simulink model "Exercise11"  (Simulink 7.2)
settings: Solver=ode45  StartTime=0.0  StopTime=2000.0  RelTol=1e-3
undefined symbols (not defined in the file): des_figposition
libraries: simeventssink1 x2, simeventsgenerators1 x2, simeventstiming1 x2, simeventsqueue1 x1, simeventsserver1 x1
settings Model: Creator=inderjot  LastModifiedBy=inderjot
settings SimEventsCC: propLogEventsScheduled=0  propLogEventsExecuted=0  propLogDepartureEvents=0  propDisplayEventCalendar=0  propDiagAttribOutput=1  propDiagFcnCallOutput=1  propDiagStatOutput=0

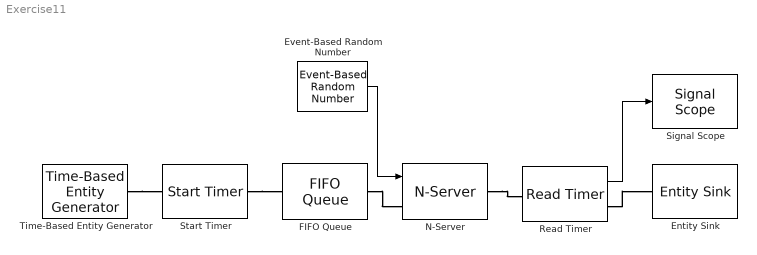
== system Exercise11 ==
  Entity Sink : simeventssink1/Entity Sink  Priority=1  SystemSampleTime=-1  AvailableForArrivals=on  StatNumberArrived=Off
  Event-Based Random Number : simeventsgenerators1/Signal Generators/Event-Based Random Number  SystemSampleTime=-1  distribution=Exponential  meanExp=5  minUnif=1  maxUnif=1  pOneBern=0.25  pSuccessBino=0.5  numTrialBino=1  meanNorm=0  stdNorm=1  minTri=1  maxTri=3  modeTri=2  thresholdLogn=0  scaleLogn=1  shapeLogn=1  pSuccessGeo=0.5  meanPoiss=1  thresholdLogl=0  scaleLogl=1  thresholdGam=0  scaleGam=1  shapeGam=1  minBeta=0  maxBeta=1  shape1Beta=1  shape2Beta=1  minUnid=0  maxUnid=1  numValueUnid=2  thresholdWbl=0  scaleWbl=1  shapeWbl=1  valueVecCont=[0 1]  cdfVecCont=[0 1]  valueVecDisc=[0 1]  probVecDisc=[0.5 0.5]  seed=9991125  IsProcessed=on  isConnected=1
  FIFO Queue : simeventsqueue1/FIFO Queue  Priority=1  SystemSampleTime=-1  Capacity=25  EnableTOPort=off  StatNumberDeparted=Off  StatNumberInBlock=Off  StatPendingEntity=Off  StatAverageWait=Off  StatAverageQueueLength=Off  StatNumberTimedout=Off
  N-Server : simeventsserver1/N-Server  Priority=1  SystemSampleTime=-1  NumberOfServers=5  ServiceTimeFrom=Signal port t  ServiceTime=1  AttributeName=ServiceTime  PriorityServiceCompletion=500  EnableTOPort=off  StatNumberDeparted=Off  StatNumberInBlock=Off  StatPendingEntity=Off  StatNumberPending=Off  StatAverageWait=Off  StatUtilization=Off  StatNumberTimedout=Off
  Read Timer : simeventstiming1/Read Timer  Priority=0  SystemSampleTime=-1  TimerTag=T1  TimerModeOption=Error  TimerStop=off  StatNumberDeparted=Off  StatTimerNumberDeparted=Off  StatTimeElapsed=Off  StatAverageTimeElapsed=On
  Signal Scope : simeventssink1/Signal Scope  Priority=1  SystemSampleTime=-1  PlotType=Continuous  InputType=Signal  NumInputs=1  AttributeNameY=Count  XInputOptionSignal=Event time  XInputOptionEntity=Event time  AttributeNameX=Count  EnableEntityOutport=on  XMin=0  XMax=2000  XLimitExceededOption=Keep axis limits unchanged  YLimitExceededOption=Stretch axis limits  AxisGrid=on  AxisLegend=off  LineDisables=""  LineColors=b  LineStyles=-  LineMarkers=.  OpenScopeAtSimStart=on  Title=Average Waiting Time in Queuing System  YLabel=Average Waiting Time  XLabel=Simulation Time  FigurePosition=des_figposition([5 60 25 25])  AxisZoom=off  DataStoreOption=Limited  DataPointsLimit=10000  StatNumberArrived=Off  ShowCountPlotted=off  ShowToolbar=on
      settings: YMin=0  YMax=6
  Start Timer : simeventstiming1/Start Timer  Priority=0  SystemSampleTime=-1  TimerTag=T1  TimerStartedOption=Warn and continue  StatNumberDeparted=Off
  Time-Based Entity Generator : simeventsgenerators1/Entity Generators/Time-Based Entity Generator  Priority=1  DialogController=des_ddg_create  DialogControllerArgs=DataTag7  SystemSampleTime=-1  GenerateEntitiesUpon=Intergeneration time from dialog  Distribution=Exponential  Minimum=0  Maximum=1  Mean=2  InitialSeed=12345  Period=1  PriorityEntityGeneration=300  GenerateEntityAtSimulationStart=on  ResponseWhenBlocked=Pause generation  ResponseWhenUnblocked=Immediate restart  EntityType=Blank  StatNumberDeparted=Off  StatPendingEntity=Off  StatAverageIntergenerationTime=Off
  wires:
  Event-Based Random Number/1 -> N-Server/1
  Read Timer/1 -> Signal Scope/1
  connections:
  FIFO Queue/RConn1 -- N-Server/LConn1
  Start Timer/RConn1 -- FIFO Queue/LConn1
  Time-Based Entity Generator/RConn1 -- Start Timer/LConn1
  N-Server/RConn1 -- Read Timer/LConn1
  Read Timer/RConn1 -- Entity Sink/LConn1
